simulink library "Trailer_Thwala_Parts"  (R2024b)
settings: Solver=VariableStepAuto  StartTime=0.0  StopTime=10.0  RelTol=1e-3
undefined symbols (not defined in the file): X, Y, Z
libraries: sm_lib x317, $bdroot x2
(part 6 of 6)

== system Trailer_Thwala_Parts/Body/Body/Exterior/A Frame/Fasteners/Nut 3 1 ==
  ReferenceFrame : sm_lib/Frames and Transforms/Reference Frame
  Solid : sm_lib/Body Elements/File Solid  ExtGeomFileName=Trailer_Thwala_Nut_3.STEP  UnitType=FromFile  ExtGeomFileUnits=m  StepReaderType=HEX  ExportConvexHullGeometry=off  InertiaType=CalculateFromGeometry  BasedOnType=Density  Density=7000  DensityUnits=kg/m^3  Mass=0.0131046920224719  MassUnits=kg  CenterOfMass=[0 2.42648642564577e-06 -2.49513273235086]  CenterOfMassUnits=mm  MomentsOfInertia=[0.434819860548486 0.434818396383243 0.592023623122136]  MomentsOfInertiaUnits=kg*mm^2  ProductsOfInertia=[6.24844514089536e-08 0 -2.62017553289772e-08]  ProductsOfInertiaUnits=kg*mm^2  GraphicType=FromGeometry  MarkerShape=Sphere  MarkerSize=10  GraphicVisPropType=SimpleVisualProperties  GraphicDiffuseColor=[0.886274509803922 0.850980392156863 0.823529411764706]  GraphicOpacity=1  GraphicSpecularColor=[0.5 0.5 0.5 1.0]  GraphicAmbientColor=[0.15 0.15 0.15 1.0]  GraphicEmissiveColor=[0.0 0.0 0.0 1.0]  GraphicShininess=75  DoExposeReferenceFrame=on  SerializedFrames=<Frames/>
  F : PMIOPort  Side=Left
  connections:
  Solid/RConn1 -- ReferenceFrame/RConn1 -- F/RConn1

== system Trailer_Thwala_Parts/Body/Body/Exterior/A Frame/Fasteners/Nut 3 2 ==
  ReferenceFrame : sm_lib/Frames and Transforms/Reference Frame
  Solid : sm_lib/Body Elements/File Solid  ExtGeomFileName=Trailer_Thwala_Nut_3.STEP  UnitType=FromFile  ExtGeomFileUnits=m  StepReaderType=HEX  ExportConvexHullGeometry=off  InertiaType=CalculateFromGeometry  BasedOnType=Density  Density=7000  DensityUnits=kg/m^3  Mass=0.0131046920224719  MassUnits=kg  CenterOfMass=[0 2.42648642564577e-06 -2.49513273235086]  CenterOfMassUnits=mm  MomentsOfInertia=[0.434819860548486 0.434818396383243 0.592023623122136]  MomentsOfInertiaUnits=kg*mm^2  ProductsOfInertia=[6.24844514089536e-08 0 -2.62017553289772e-08]  ProductsOfInertiaUnits=kg*mm^2  GraphicType=FromGeometry  MarkerShape=Sphere  MarkerSize=10  GraphicVisPropType=SimpleVisualProperties  GraphicDiffuseColor=[0.886274509803922 0.850980392156863 0.823529411764706]  GraphicOpacity=1  GraphicSpecularColor=[0.5 0.5 0.5 1.0]  GraphicAmbientColor=[0.15 0.15 0.15 1.0]  GraphicEmissiveColor=[0.0 0.0 0.0 1.0]  GraphicShininess=75  DoExposeReferenceFrame=on  SerializedFrames=<Frames/>
  F : PMIOPort  Side=Left
  connections:
  Solid/RConn1 -- ReferenceFrame/RConn1 -- F/RConn1

== system Trailer_Thwala_Parts/Body/Body/Exterior/A Frame/Fasteners/Washer_1_2_RIGID ==
  ReferenceFrame : sm_lib/Frames and Transforms/Reference Frame
  Solid : sm_lib/Body Elements/File Solid  ExtGeomFileName=Trailer_Thwala_AFrame_Washer.STEP  UnitType=FromFile  ExtGeomFileUnits=m  StepReaderType=HEX  ExportConvexHullGeometry=off  InertiaType=CalculateFromGeometry  BasedOnType=Density  Density=7000  DensityUnits=kg/m^3  Mass=0.00350456441480393  MassUnits=kg  CenterOfMass=[-1.00000000000001 0 0]  CenterOfMassUnits=mm  MomentsOfInertia=[0.223525499081713 0.112930937679123 0.112930937679123]  MomentsOfInertiaUnits=kg*mm^2  ProductsOfInertia=[0 0 0]  ProductsOfInertiaUnits=kg*mm^2  GraphicType=FromGeometry  MarkerShape=Sphere  MarkerSize=10  GraphicVisPropType=SimpleVisualProperties  GraphicDiffuseColor=[0.886274509803922 0.850980392156863 0.823529411764706]  GraphicOpacity=1  GraphicSpecularColor=[0.5 0.5 0.5 1.0]  GraphicAmbientColor=[0.15 0.15 0.15 1.0]  GraphicEmissiveColor=[0.0 0.0 0.0 1.0]  GraphicShininess=75  DoExposeReferenceFrame=on  SerializedFrames=<Frames/>
  F : PMIOPort  Side=Left
  connections:
  Solid/RConn1 -- ReferenceFrame/RConn1 -- F/RConn1

== system Trailer_Thwala_Parts/Body/Body/Exterior/A Frame/Fasteners/Washer_1_3_RIGID ==
  ReferenceFrame : sm_lib/Frames and Transforms/Reference Frame
  Solid : sm_lib/Body Elements/File Solid  ExtGeomFileName=Trailer_Thwala_AFrame_Washer.STEP  UnitType=FromFile  ExtGeomFileUnits=m  StepReaderType=HEX  ExportConvexHullGeometry=off  InertiaType=CalculateFromGeometry  BasedOnType=Density  Density=7000  DensityUnits=kg/m^3  Mass=0.00350456441480393  MassUnits=kg  CenterOfMass=[-1.00000000000001 0 0]  CenterOfMassUnits=mm  MomentsOfInertia=[0.223525499081713 0.112930937679123 0.112930937679123]  MomentsOfInertiaUnits=kg*mm^2  ProductsOfInertia=[0 0 0]  ProductsOfInertiaUnits=kg*mm^2  GraphicType=FromGeometry  MarkerShape=Sphere  MarkerSize=10  GraphicVisPropType=SimpleVisualProperties  GraphicDiffuseColor=[0.886274509803922 0.850980392156863 0.823529411764706]  GraphicOpacity=1  GraphicSpecularColor=[0.5 0.5 0.5 1.0]  GraphicAmbientColor=[0.15 0.15 0.15 1.0]  GraphicEmissiveColor=[0.0 0.0 0.0 1.0]  GraphicShininess=75  DoExposeReferenceFrame=on  SerializedFrames=<Frames/>
  F : PMIOPort  Side=Left
  connections:
  Solid/RConn1 -- ReferenceFrame/RConn1 -- F/RConn1

== system Trailer_Thwala_Parts/Body/Body/Exterior/A Frame/Fasteners/Washer_1_4_RIGID ==
  ReferenceFrame : sm_lib/Frames and Transforms/Reference Frame
  Solid : sm_lib/Body Elements/File Solid  ExtGeomFileName=Trailer_Thwala_AFrame_Washer.STEP  UnitType=FromFile  ExtGeomFileUnits=m  StepReaderType=HEX  ExportConvexHullGeometry=off  InertiaType=CalculateFromGeometry  BasedOnType=Density  Density=7000  DensityUnits=kg/m^3  Mass=0.00350456441480393  MassUnits=kg  CenterOfMass=[-1.00000000000001 0 0]  CenterOfMassUnits=mm  MomentsOfInertia=[0.223525499081713 0.112930937679123 0.112930937679123]  MomentsOfInertiaUnits=kg*mm^2  ProductsOfInertia=[0 0 0]  ProductsOfInertiaUnits=kg*mm^2  GraphicType=FromGeometry  MarkerShape=Sphere  MarkerSize=10  GraphicVisPropType=SimpleVisualProperties  GraphicDiffuseColor=[0.886274509803922 0.850980392156863 0.823529411764706]  GraphicOpacity=1  GraphicSpecularColor=[0.5 0.5 0.5 1.0]  GraphicAmbientColor=[0.15 0.15 0.15 1.0]  GraphicEmissiveColor=[0.0 0.0 0.0 1.0]  GraphicShininess=75  DoExposeReferenceFrame=on  SerializedFrames=<Frames/>
  F : PMIOPort  Side=Left
  connections:
  Solid/RConn1 -- ReferenceFrame/RConn1 -- F/RConn1
